simulink model "ClosedLoop_Kcont_2015a"  (Simulink 8.5)
settings: Solver=ode4  SolverMode=SingleTasking  StartTime=0.0  StopTime=10  FixedStep=0.001  RelTol=1e-3
undefined symbols (not defined in the file): theta0, x0
settings Model: Creator=manzand  LastModifiedBy=dieman95  CovMetricSettings=dwe  CovHtmlReporting=off  covSaveCumulativeToWorkspaceVar=off  CovSaveSingleToWorkspaceVar=off  CovExternalEMLEnable=on
settings DataIOCC: LimitDataPoints=off  SaveFormat=Dataset  SignalLoggingSaveFormat=Dataset
settings OptimizationCC: ExpressionDepthLimit=128
settings DebuggingCC: UnderspecifiedInitializationDetection=Simplified  MergeDetectMultiDrivingBlocksExec=error  FcnCallInpInsideContextMsg=EnableAllAsError  StateNameClashWarn=none  SFUnexpectedBacktrackingDiag=error  SFNoUnconditionalDefaultTransitionDiag=error
settings HardwareCC: ProdBitPerPointer=64  ProdLargestAtomicFloat=Float  ProdIntDivRoundTo=Zero  ProdEndianess=LittleEndian  ProdHWDeviceType=Specified
settings ModelReferenceCC: PropagateSignalLabelsOutOfModel=on
settings GRTTargetCC: TargetLangStandard=C99 (ISO)  GeneratePreprocessorConditionals=Use local settings  CombineOutputUpdateFcns=on  GRTInterface=off

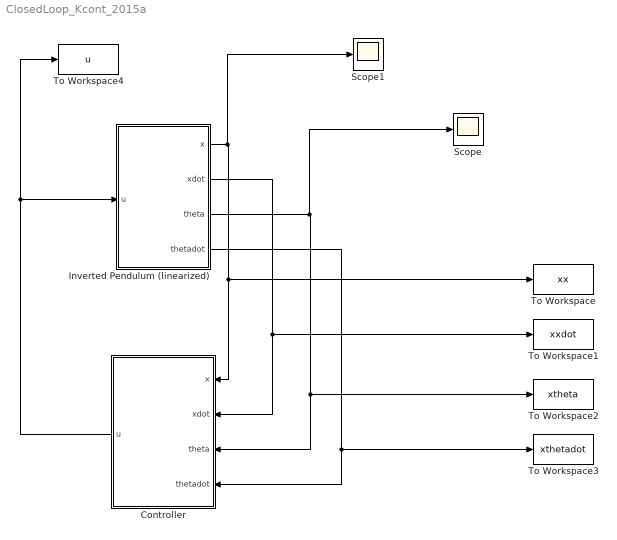
== system ClosedLoop_Kcont_2015a ==
  Controller : Subsystem
  Inverted Pendulum (linearized) : Subsystem
  Scope : Scope
      settings: TimeRange=auto  MaxDataPoints=5000  SaveToWorkspace=off  SaveName=ScopeData  YMin=-0.09575  YMax=0.12175  SampleTime=-1
  Scope1 : Scope
      settings: TimeRange=auto  MaxDataPoints=5000  SaveToWorkspace=off  YMin=-0.06984  YMax=0.68893  SampleTime=-1
  To Workspace : ToWorkspace  VariableName=xx  SampleTime=0.005
      settings: Decimation=2  Save2DSignal=2-D array (concatenate along first dimension)
  To Workspace1 : ToWorkspace  VariableName=xxdot  SampleTime=0.005
      settings: Decimation=2  Save2DSignal=2-D array (concatenate along first dimension)
  To Workspace2 : ToWorkspace  VariableName=xtheta  SampleTime=0.005
      settings: Decimation=2  Save2DSignal=2-D array (concatenate along first dimension)
  To Workspace3 : ToWorkspace  VariableName=xthetadot  SampleTime=0.005
      settings: Decimation=2  Save2DSignal=2-D array (concatenate along first dimension)
  To Workspace4 : ToWorkspace  VariableName=u  SampleTime=0.005
      settings: Decimation=2  Save2DSignal=2-D array (concatenate along first dimension)
  wires:
  Inverted Pendulum (linearized)/1(x) -> Scope1/1, To Workspace/1, Controller/1(x)
  Inverted Pendulum (linearized)/2(xdot) -> To Workspace1/1, Controller/2(xdot)
  Inverted Pendulum (linearized)/3(theta) -> Scope/1, To Workspace2/1, Controller/3(theta)
  Inverted Pendulum (linearized)/4(thetadot) -> To Workspace3/1, Controller/4(thetadot)
  Controller/1(u) -> To Workspace4/1, Inverted Pendulum (linearized)/1(u)

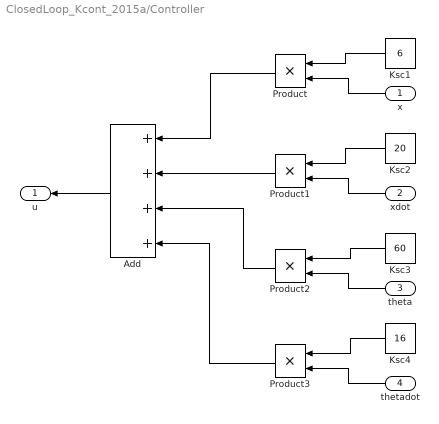
== system ClosedLoop_Kcont_2015a/Controller ==
  x : Inport
  xdot : Inport  Port=2
  theta : Inport  Port=3
  thetadot : Inport  Port=4
  Add : Sum  Inputs=++++
  Ksc1 : Constant  Value=6
  Ksc2 : Constant  Value=20
  Ksc3 : Constant  Value=60
  Ksc4 : Constant  Value=16
  Product{,1..3} (4 alike) : Product
  u : Outport
  wires:
  Product1/1 -> Add/2
  Add/1 -> u/1
  Product2/1 -> Add/3
  Product3/1 -> Add/4
  Product/1 -> Add/1
  Ksc3/1 -> Product2/1
  thetadot/1 -> Product3/2
  x/1 -> Product/2
  Ksc2/1 -> Product1/1
  xdot/1 -> Product1/2
  Ksc1/1 -> Product/1
  Ksc4/1 -> Product3/1
  theta/1 -> Product2/2

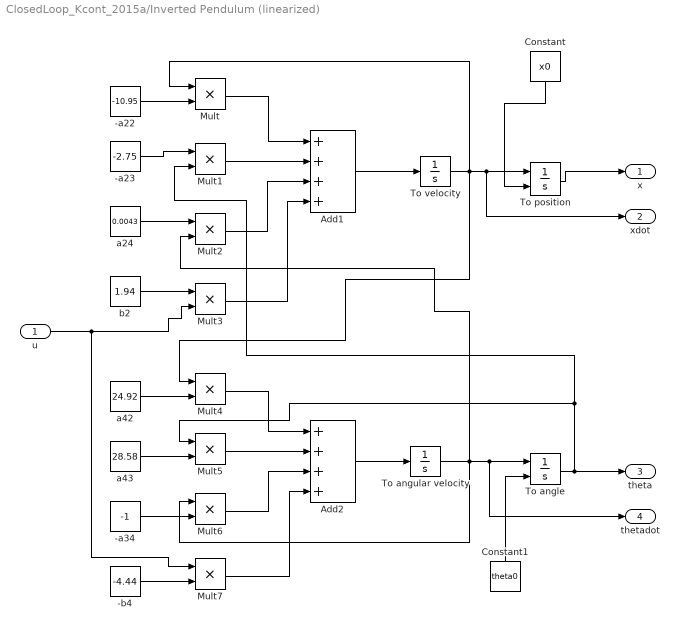
== system ClosedLoop_Kcont_2015a/Inverted Pendulum (linearized) ==
  u : Inport
  -a22 : Constant  Value=-10.95
  -a23 : Constant  Value=-2.75
  -a34 : Constant  Value=-1
  -b4 : Constant  Value=-4.44
  Add1 : Sum  Inputs=++++
  Add2 : Sum  Inputs=++++
  Constant : Constant  Value=x0
  Constant1 : Constant  Value=theta0
  Mult{,1..7} (8 alike) : Product  Inputs=**
  To angle : Integrator  InitialConditionSource=external  InitialCondition=1.5
  To angular velocity : Integrator
  To position : Integrator  InitialConditionSource=external  InitialCondition=1
  To velocity : Integrator
  a24 : Constant  Value=0.0043
  a42 : Constant  Value=24.92
  a43 : Constant  Value=28.58
  b2 : Constant  Value=1.94
  x : Outport
  xdot : Outport  Port=2
  theta : Outport  Port=3
  thetadot : Outport  Port=4
  wires:
  -a22/1 -> Mult/2
  Add2/1 -> To angular velocity/1
  -a34/1 -> Mult6/2
  -b4/1 -> Mult7/2
  Mult6/1 -> Add2/3
  Mult3/1 -> Add1/4
  Mult1/1 -> Add1/2
  Add1/1 -> To velocity/1
  b2/1 -> Mult3/1
  To angular velocity/1 -> Mult6/1, Mult2/2, thetadot/1, To angle/1
  -a23/1 -> Mult1/1
  To velocity/1 -> Mult4/1, Mult/1, xdot/1, To position/1
  To angle/1 -> theta/1, Mult5/1, Mult1/2
  Mult7/1 -> Add2/4
  a43/1 -> Mult5/2
  Mult4/1 -> Add2/1
  Mult2/1 -> Add1/3
  u/1 -> Mult7/1, Mult3/2
  a42/1 -> Mult4/2
  Mult/1 -> Add1/1
  Mult5/1 -> Add2/2
  a24/1 -> Mult2/1
  To position/1 -> x/1
  Constant1/1 -> To angle/2
  Constant/1 -> To position/2
